simulink model "rolltesting"  (R2019a)
settings: Solver=VariableStepAuto  StartTime=0.0  StopTime=3  RelTol=1e-3
values from neighbouring files (symbols this model uses):
  D = zeros(size(B))    [RocketOutputFunction.m]    (also in StateSpaceController.m = zeros(13, 3); TimeDelayCompensationElevator.m = [0; 0])
  F = eye(6)    [MEKFAttitudeOnly.m]
  Ki2 = lqr(Ai2, Bi2, Q, R)    [StateSpaceController.m]
  q = x(13:16)    [AdaptiveLQR.m]    (also in MEKF.m = nominal_state(4:7); MEKFAttitudeOnly.m = [1 0 0 0]; MEKF_old.m = nominal_state(4:7); NonlinearStateEstimationForActuatorDelay.m = x(4:7))
  r = sym('r', [3 1])    [StateSpaceController.m]    (also in TimeDelayCompensationElevator.m = [0;0]; Tracker.m = [0; 0; -(rocket_length - Average_cg)])
  s = linspace(0, 100, nums)    [ImpactVelocityFunction.m]    (also in ImpactVelocityNotParallelMatlab.m = 1:5:500; ParallelImpactVelocity.m = .1:.01:500; ParralelRun.m = linspace(5,7, nums); RunImpactVelocityParforCompiled.m = 1:0.1:500)
undefined symbols (not defined in the file or in its folder): deg, e0_0, e1_0, e2_0, e3_0, Earth, Light, magnitude, MIL, rad, WGS84
libraries: aerolibutil x9, aerolibconvert2 x4, simulink x3, sharedtransform x3, aerolibwind2 x3, aerolibfltsims x2, aerolibasang x2, aerolibatmos2 x1, aerolibbdyn x1, aerolibtransform2 x1
settings Model: Creator=rag  LastModifiedBy=rag

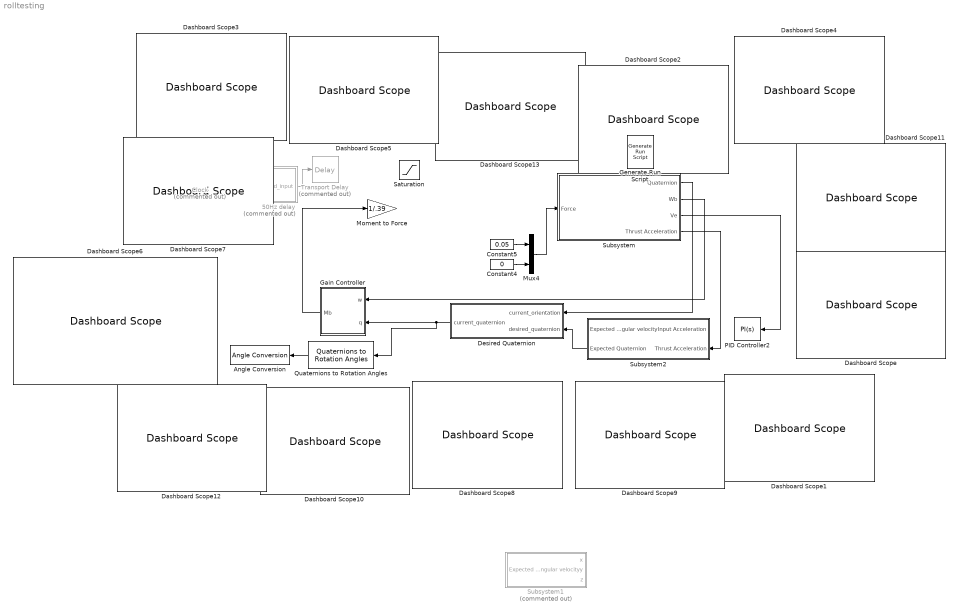
== system rolltesting ==
  50Hz delay : MATLAB Function  Commented=on  TreatAsAtomicUnit=on
  Angle Conversion : aerolibconvert2/Angle Conversion  IU=rad  OU=deg
  Clock : Clock  Commented=on
      settings: Decimation=100
  Constant4 : Constant  Value=0
  Constant5 : Constant  Value=0.05
  Dashboard Scope{,1..13} (14 alike) : DashboardScope
  Desired Quaternion : MATLAB Function  TreatAsAtomicUnit=on
  Gain Controller : Subsystem
  Generate Run Script : aerolibfltsims/Generate Run Script  Architecture=Win64  dataFlow=Send  GeometryModelName=Rocket  AirportId=PHNL  RunwayId=04L  InitialAltitude=13  InitialHeading=0  OffsetDistance=0  OffsetAzimuth=0  InstallScenery=off  DisableShaders=off  OriginAddress=127.0.0.1  DestinationPort=5502  OriginPort=5505  LocalAddress=127.0.0.1  OutputFileName=runfg.bat  FlightGearBaseDirectory=C:\Program Files\FlightGear 2018.2.2
  Moment to Force : Gain  Gain=1/.39
  Mux4 : Mux  Inputs=2
  PID Controller2 : simulink/Continuous/PID Controller  Controller=PI  Form=Parallel  TimeDomain=Continuous-time  SampleTime=-1  IntegratorMethod=Forward Euler  FilterMethod=Forward Euler  ControllerParametersSource=internal  P=-0.4  I=-0.3  D=0  UseFilter=on  N=100  TunerSelectOption=Transfer Function Based (PID Tuner App)  InitialConditionSource=internal  InitialConditionForIntegrator=0  InitialConditionForFilter=0  DifferentiatorICPrevScaledInput=0  ExternalReset=none  TrackingMode=off  Kt=1  LimitOutput=off  UpperSaturationLimit=inf  LowerSaturationLimit=-inf  LinearizeAsGain=on  AntiWindupMode=none  Kb=1  POutMin=[]  POutMax=[]  IOutMin=[]  IOutMax=[]  DOutMin=[]  DOutMax=[]  NOutMin=[]  NOutMax=[]  SumOutMin=[]  SumOutMax=[]  SaturationOutMin=[]  SaturationOutMax=[]  PParamMin=[]  PParamMax=[]  IParamMin=[]  IParamMax=[]  DParamMin=[]  DParamMax=[]  NParamMin=[]  NParamMax=[]  KbParamMin=[]  KbParamMax=[]  KtParamMin=[]  KtParamMax=[]  KbOutMin=[]  KbOutMax=[]  KtOutMin=[]  KtOutMax=[]  IntegratorOutMin=[]  IntegratorOutMax=[]  FilterOutMin=[]  FilterOutMax=[]  SumI1OutMin=[]  SumI1OutMax=[]  SumI2OutMin=[]  SumI2OutMax=[]  SumI3OutMin=[]  SumI3OutMax=[]  SumI4OutMin=[]  SumI4OutMax=[]  SumDOutMin=[]  SumDOutMax=[]  DifferentiatorOutMin=[]  DifferentiatorOutMax=[]  FilterDiffOutCoefMin=[]  FilterDiffOutCoefMax=[]  ReciprocalOutMin=[]  ReciprocalOutMax=[]  SumDenOutMin=[]  SumDenOutMax=[]  SumNumOutMin=[]  SumNumOutMax=[]  DivideOutMin=[]  DivideOutMax=[]  IntegratorContinuousStateAttributes=''  IntegratorStateMustResolveToSignalObject=off  IntegratorRTWStateStorageClass=Auto  FilterContinuousStateAttributes=''  FilterStateMustResolveToSignalObject=off  FilterRTWStateStorageClass=Auto  ParallelPVariant=InternalParameters  IdealPVariant=Disabled  IVariant=InternalParameters  DVariant=Disabled  IntegratorVariant=Continuous  SatVariant=Disabled  AWVariant=Passthrough  PCopyVariant=Disabled  TRVariant=Disabled  FdbkBlocksVariant=Forward  IdealPFdbkVariant=Disabled  SatFdbkVariant=Disabled  DerivativeFilterVariant=Disabled  NVariant=Disabled  NCopyVariant=Disabled_SignalSpec  FilterICVariant=Disabled  IntegratorICVariant=InternalICs  ExternalResetVariant=Disabled  TRSumVariant=Passthrough  SumFdbkVariant=Disabled  SumVariant=Sum_PI
  Quaternions to Rotation Angles : sharedtransform/Quaternions to Rotation Angles  rotationOrder=XYZ  aMode=aMode
      settings: SourceProductBaseCode=AE
  Saturation : Saturate  UpperLimit=1.5  LowerLimit=-1.5
  Subsystem : Subsystem
  Subsystem1 : Subsystem  Commented=on
  Subsystem2 : Subsystem
  Transport Delay : TransportDelay  Commented=on  DelayTime=0.015  TransDelayFeedthrough=on
  wires:
  Quaternions to Rotation Angles/1 -> Angle Conversion/1
  Desired Quaternion/1(current_quaternion) -> Quaternions to Rotation Angles/1, Gain Controller/2(q)
  Gain Controller/1(Mb) -> Moment to Force/1
  Subsystem/4(Thrust Acceleration) -> Subsystem2/2(Thrust Acceleration)
  50Hz delay/1(delayed_input) -> Transport Delay/1
  Subsystem/3(Ve) -> PID Controller2/1
  Subsystem/2(Wb) -> Gain Controller/1(w)
  Subsystem2/2(Expected Quaternion) -> Desired Quaternion/2(desired_quaternion)
  Clock/1 -> 50Hz delay/1(time)
  Subsystem/1(Quaternion) -> Desired Quaternion/1(current_orientation)
  Mux4/1 -> Subsystem/1(Force)
  Constant5/1 -> Mux4/1
  Constant4/1 -> Mux4/2

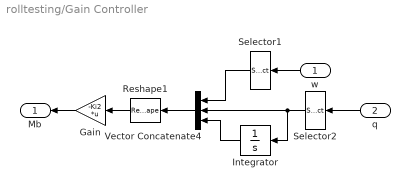
== system rolltesting/Gain Controller ==
  w : Inport
  q : Inport  Port=2
  Gain : Gain  Gain=-Ki2  Multiplication=Matrix(K*u)
  Integrator : Integrator
  Reshape1 : Reshape  OutputDimensionality=Column vector (2-D)
  Selector1 : Selector  InputPortWidth=3  IndexOptions=Index vector (dialog)  Indices=[2 1]  OutputSizes=1
  Selector2 : Selector  InputPortWidth=4  IndexOptions=Index vector (dialog)  Indices=[3 2]  OutputSizes=1
  Vector Concatenate4 : Concatenate  NumInputs=3
  Mb : Outport
  wires:
  Vector Concatenate4/1 -> Reshape1/1
  Reshape1/1 -> Gain/1
  Selector2/1 -> Integrator/1, Vector Concatenate4/2
  Integrator/1 -> Vector Concatenate4/3
  q/1 -> Selector2/1
  Gain/1 -> Mb/1
  Selector1/1 -> Vector Concatenate4/1
  w/1 -> Selector1/1

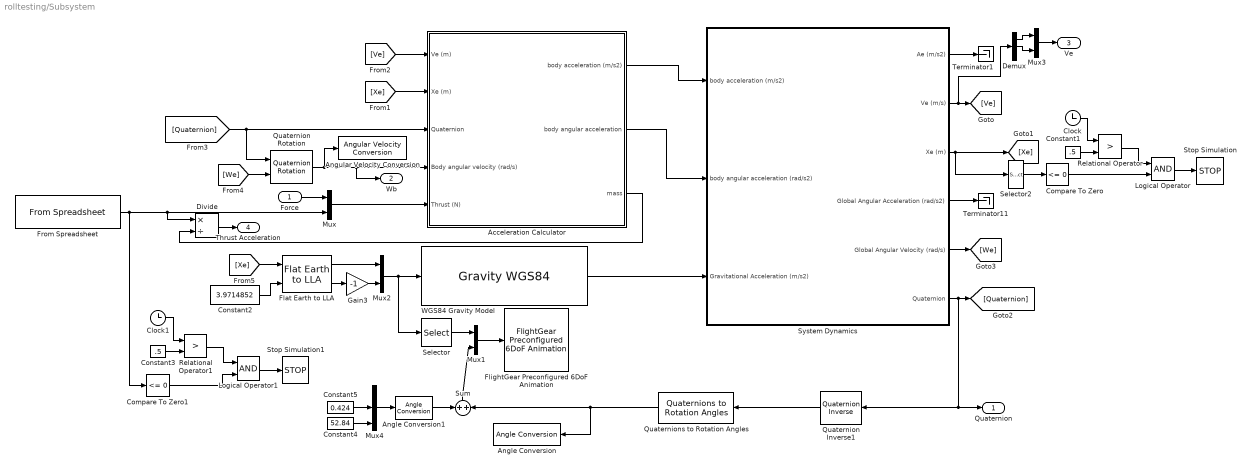
== system rolltesting/Subsystem ==
  Force : Inport  PortDimensions=2
  Acceleration Calculator : Subsystem
  Angle Conversion : aerolibconvert2/Angle Conversion  IU=rad  OU=deg
  Angle Conversion1 : aerolibconvert2/Angle Conversion  IU=deg  OU=rad
  Angular Velocity Conversion : aerolibconvert2/Angular Velocity Conversion  IU=rad/s  OU=deg/s
      settings: SourceProductName=Aerospace Blockset
  Clock : Clock
  Clock1 : Clock
  Compare To Zero : simulink/Logic and Bit Operations/Compare To Zero  relop=<=  OutDataTypeStr=boolean
  Compare To Zero1 : simulink/Logic and Bit Operations/Compare To Zero  relop=<=  OutDataTypeStr=boolean
  Constant1 : Constant  Value=.5
  Constant2 : Constant  Value=3.9714852
  Constant3 : Constant  Value=.5
  Constant4 : Constant  Value=52.84
  Constant5 : Constant  Value=0.424
  Demux : Demux  Outputs=3
  Divide : Product  Inputs=*/
  Flat Earth to LLA : aerolibtransform2/Flat Earth to LLA  units=Metric (MKS)  ptype=Earth (WGS84)  F=1/298.257223563  R=6378137  LL0=[21.318358277648 -157.9232805920725]  psi=052
  FlightGear Preconfigured 6DoF Animation : aerolibfltsims/FlightGear Preconfigured 6DoF Animation  xFlightGearVersion=v2018.2  DestinationIpAddress=127.0.0.1  DestinationPort=5502  SampleTime=1/100  packetVersion=24
      settings: SourceProductName=Aerospace Blockset
  From Spreadsheet : FromSpreadsheet  FileName=F10_Thrust.xls  Range=A1:B29  ExtrapolationBeforeFirstDataPoint=Hold first value  ExtrapolationAfterLastDataPoint=Hold last value
  Gain3 : Gain  Gain=-1
  Logical Operator : Logic  AllPortsSameDT=off  OutDataTypeStr=boolean
  Logical Operator1 : Logic  AllPortsSameDT=off  OutDataTypeStr=boolean
  Mux{,1..3} (4 alike) : Mux  Inputs=2
  Mux4 : Mux  Inputs=3
  Quaternion Inverse1 : aerolibutil/Quaternion Inverse
      settings: SourceProductName=Aerospace Blockset
  Quaternion Rotation : aerolibutil/Quaternion Rotation
  Quaternions to Rotation Angles : sharedtransform/Quaternions to Rotation Angles  rotationOrder=XYZ  aMode=aMode
      settings: SourceProductBaseCode=AE
  Relational Operator : RelationalOperator  Operator=>  OutDataTypeStr=boolean  RndMeth=Simplest
  Relational Operator1 : RelationalOperator  Operator=>  OutDataTypeStr=boolean  RndMeth=Simplest
  Selector : Selector  InputPortWidth=3  IndexOptions=Index vector (dialog)  Indices=[2 1 3]  OutputSizes=1
  Selector2 : Selector  InputPortWidth=3  IndexOptions=Index vector (dialog)  Indices=[3]  OutputSizes=1
  Stop Simulation : Stop
  Stop Simulation1 : Stop
  Sum : Sum
  System Dynamics : Subsystem
  Terminator1 : Terminator
  Terminator11 : Terminator
  "WGS84 Gravity Model  " : GravityWGS84
  Quaternion : Outport
  Wb : Outport  Port=2
  Ve : Outport  Port=3
  Thrust Acceleration : Outport  Port=4
  wires:
  System Dynamics/5(Global Angular Velocity (rad/s)) -> [We]
  Selector/1 -> Mux1/1
  [Quaternion] -> Quaternion Rotation/1, Acceleration Calculator/3(Quaternion)
  Flat Earth to LLA/1 -> Mux2/1
  Flat Earth to LLA/2 -> Gain3/1
  Mux/1 -> Acceleration Calculator/5(Thrust (N))
  Gain3/1 -> Mux2/2
  Quaternions to Rotation Angles/1 -> Sum/2, Angle Conversion/1
  Mux2/1 -> Selector/1, "WGS84 Gravity Model  "/1
  System Dynamics/2(Ve (m/s)) -> Demux/1, [Ve]
  Constant2/1 -> Flat Earth to LLA/2
  Acceleration Calculator/1(body acceleration (m/s2)) -> System Dynamics/1(body acceleration (m/s2))
  System Dynamics/6(Quaternion) -> Quaternion Inverse1/1, Quaternion/1, [Quaternion]
  From Spreadsheet/1 -> Compare To Zero1/1, Divide/1, Mux/2
  Quaternion Rotation/1 -> Angular Velocity Conversion/1, Wb/1, Acceleration Calculator/4(Body angular velocity (rad/s))
  [We] -> Quaternion Rotation/2
  [Ve] -> Acceleration Calculator/1(Ve (m))
  Mux1/1 -> FlightGear Preconfigured 6DoF Animation/1
  "WGS84 Gravity Model  "/1 -> System Dynamics/3(Gravitational Acceleration (m/s2))
  [Xe] -> Acceleration Calculator/2(Xe (m))
  Force/1 -> Mux/1
  System Dynamics/1(Ae (m/s2)) -> Terminator1/1
  System Dynamics/4(Global Angular Acceleration (rad/s2)) -> Terminator11/1
  Clock/1 -> Relational Operator/1
  Compare To Zero/1 -> Logical Operator/2
  Logical Operator/1 -> Stop Simulation/1
  Relational Operator/1 -> Logical Operator/1
  Constant1/1 -> Relational Operator/2
  Selector2/1 -> Compare To Zero/1
  Relational Operator1/1 -> Logical Operator1/1
  Logical Operator1/1 -> Stop Simulation1/1
  Constant3/1 -> Relational Operator1/2
  Clock1/1 -> Relational Operator1/1
  Compare To Zero1/1 -> Logical Operator1/2
  Demux/1 -> Mux3/1
  Demux/2 -> Mux3/2
  Mux3/1 -> Ve/1
  Constant4/1 -> Mux4/3
  Mux4/1 -> Angle Conversion1/1
  Constant5/1 -> Mux4/2
  Angle Conversion1/1 -> Sum/1
  [Xe] -> Flat Earth to LLA/1
  Sum/1 -> Mux1/2
  System Dynamics/3(Xe (m)) -> [Xe], Selector2/1
  Quaternion Inverse1/1 -> Quaternions to Rotation Angles/1
  Acceleration Calculator/3(mass) -> Divide/2
  Divide/1 -> Thrust Acceleration/1
  Acceleration Calculator/2(body angular acceleration) -> System Dynamics/2(body angular acceleration (rad/s2))

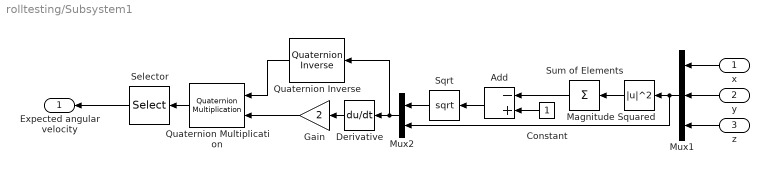
== system rolltesting/Subsystem1 ==
  x : Inport
  y : Inport  Port=2
  z : Inport  Port=3
  Add : Sum  Inputs=-+
  Constant : Constant
  Derivative : Derivative
  Gain : Gain  Gain=2
  Magnitude Squared : Math  Operator=magnitude^2  SaturateOnIntegerOverflow=on
  Mux1 : Mux  Inputs=3
  Mux2 : Mux  Inputs=2
  Quaternion Inverse : aerolibutil/Quaternion Inverse
      settings: SourceProductName=Aerospace Blockset
  Quaternion Multiplication : aerolibutil/Quaternion Multiplication
  Selector : Selector  InputPortWidth=4  IndexOptions=Index vector (dialog)  Indices=[2 3 4]  OutputSizes=1
  Sqrt : Sqrt  SaturateOnIntegerOverflow=on
  Sum of Elements : Sum  Inputs=+
  Expected angular velocity : Outport
  wires:
  Quaternion Inverse/1 -> Quaternion Multiplication/1
  x/1 -> Mux1/1
  Gain/1 -> Quaternion Multiplication/2
  Magnitude Squared/1 -> Sum of Elements/1
  Add/1 -> Sqrt/1
  Mux1/1 -> Mux2/2, Magnitude Squared/1
  Quaternion Multiplication/1 -> Selector/1
  Mux2/1 -> Quaternion Inverse/1, Derivative/1
  Constant/1 -> Add/2
  Derivative/1 -> Gain/1
  Sqrt/1 -> Mux2/1
  z/1 -> Mux1/3
  y/1 -> Mux1/2
  Sum of Elements/1 -> Add/1
  Selector/1 -> Expected angular velocity/1

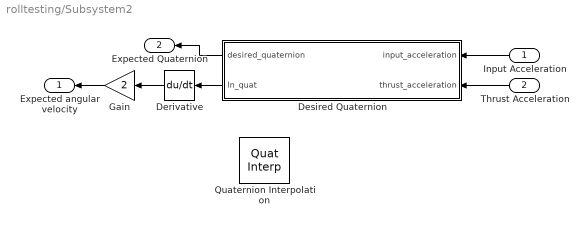
== system rolltesting/Subsystem2 ==
  Input Acceleration : Inport  PortDimensions=[2]
  Thrust Acceleration : Inport  Port=2
  Derivative : Derivative
  Desired Quaternion : MATLAB Function  TreatAsAtomicUnit=on
  Gain : Gain  Gain=2
  Quaternion Interpolation : QuatInterp
  Expected angular velocity : Outport
  Expected Quaternion : Outport  Port=2
  wires:
  Thrust Acceleration/1 -> Desired Quaternion/2(thrust_acceleration)
  Gain/1 -> Expected angular velocity/1
  Desired Quaternion/1(desired_quaternion) -> Expected Quaternion/1
  Input Acceleration/1 -> Desired Quaternion/1(input_acceleration)
  Derivative/1 -> Gain/1
  Desired Quaternion/2(ln_quat) -> Derivative/1

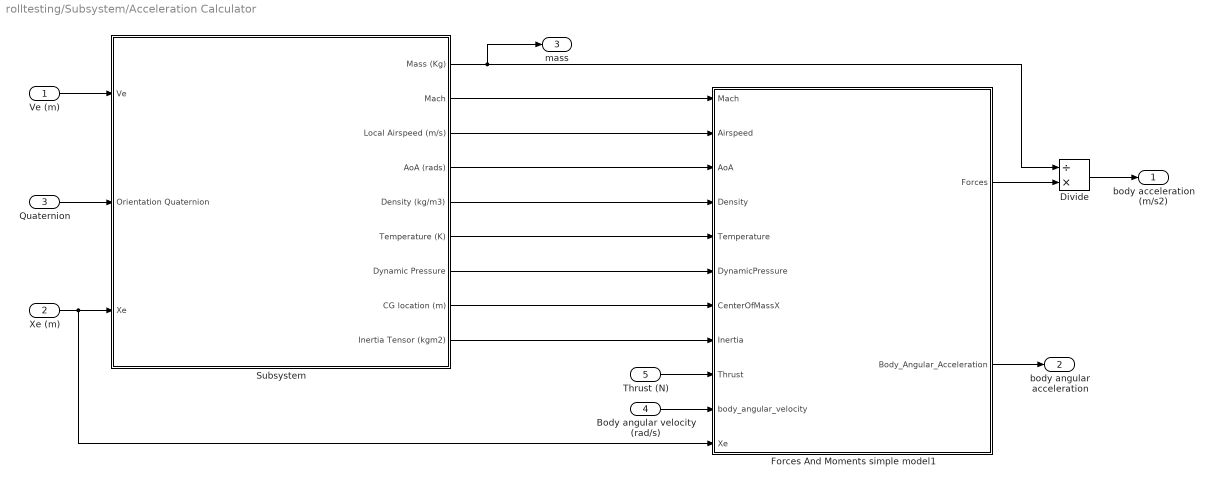
== system rolltesting/Subsystem/Acceleration Calculator ==
  Ve (m) : Inport
  Xe (m) : Inport  Port=2
  Quaternion : Inport  Port=3
  Body angular velocity (rad/s) : Inport  Port=4
  Thrust (N) : Inport  Port=5
  Divide : Product  Inputs=/*
  Forces And Moments simple model1 : MATLAB Function  TreatAsAtomicUnit=on
  Subsystem : Subsystem
  body acceleration (m/s2) : Outport
  body angular acceleration : Outport  Port=2
  mass : Outport  Port=3
  wires:
  Subsystem/4(AoA (rads)) -> Forces And Moments simple model1/3(AoA)
  Xe (m)/1 -> Forces And Moments simple model1/11(Xe), Subsystem/3(Xe)
  Subsystem/6(Temperature (K)) -> Forces And Moments simple model1/5(Temperature)
  Subsystem/8(CG location (m)) -> Forces And Moments simple model1/7(CenterOfMassX)
  Subsystem/3(Local Airspeed (m/s)) -> Forces And Moments simple model1/2(Airspeed)
  Subsystem/7(Dynamic Pressure) -> Forces And Moments simple model1/6(DynamicPressure)
  Subsystem/2(Mach) -> Forces And Moments simple model1/1(Mach)
  Subsystem/5(Density (kg/m3)) -> Forces And Moments simple model1/4(Density)
  Thrust (N)/1 -> Forces And Moments simple model1/9(Thrust)
  Forces And Moments simple model1/1(Forces) -> Divide/2
  Body angular velocity (rad/s)/1 -> Forces And Moments simple model1/10(body_angular_velocity)
  Ve (m)/1 -> Subsystem/1(Ve)
  Quaternion/1 -> Subsystem/2(Orientation Quaternion)
  Subsystem/9(Inertia Tensor (kgm2)) -> Forces And Moments simple model1/8(Inertia)
  Forces And Moments simple model1/2(Body_Angular_Acceleration) -> body angular acceleration/1
  Divide/1 -> body acceleration (m/s2)/1
  Subsystem/1(Mass (Kg)) -> mass/1, Divide/1

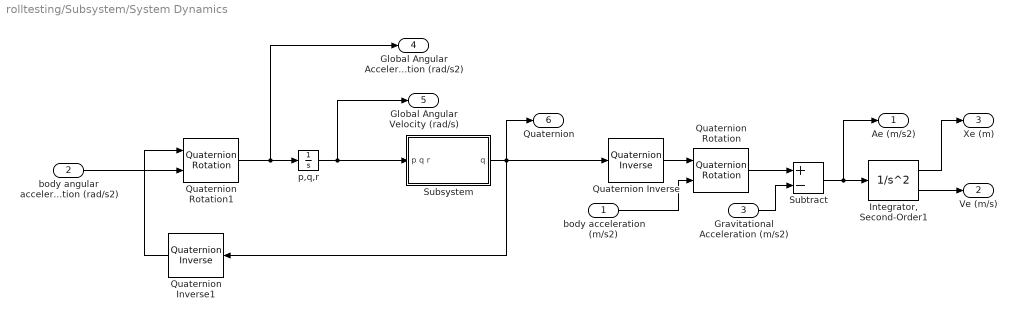
== system rolltesting/Subsystem/System Dynamics ==
  body acceleration (m/s2) : Inport  Unit=N*m  PortDimensions=3
  body angular acceleration (rad/s2) : Inport  Port=2  PortDimensions=3
  Gravitational Acceleration (m/s2) : Inport  Port=3
  "Integrator, Second-Order1" : SecondOrderIntegrator  LimitX=on  LowerLimitX=[-inf; -inf; 0]
  Quaternion Inverse : aerolibutil/Quaternion Inverse
      settings: SourceProductName=Aerospace Blockset
  Quaternion Inverse1 : aerolibutil/Quaternion Inverse
      settings: SourceProductName=Aerospace Blockset
  Quaternion Rotation : aerolibutil/Quaternion Rotation
  Quaternion Rotation1 : aerolibutil/Quaternion Rotation
  Subsystem : Subsystem
  Subtract : Sum  Inputs=+-
  "p,q,r " : Integrator
  Ae (m/s2) : Outport  Unit=m/s^2
  Ve (m/s) : Outport  Port=2  Unit=m/s
  Xe (m) : Outport  Port=3  Unit=m
  Global Angular Acceleration (rad/s2) : Outport  Port=4  Unit=rad/s
  Global Angular Velocity (rad/s) : Outport  Port=5  Unit=rad/s
  Quaternion : Outport  Port=6  Unit=1
  wires:
  "p,q,r "/1 -> Subsystem/1(p q r), Global Angular Velocity (rad/s)/1
  body acceleration (m/s2)/1 -> Quaternion Rotation/2
  Subsystem/1(q) -> Quaternion/1, Quaternion Inverse/1, Quaternion Inverse1/1
  Quaternion Inverse/1 -> Quaternion Rotation/1
  "Integrator, Second-Order1"/1 -> Xe (m)/1
  Gravitational Acceleration (m/s2)/1 -> Subtract/2
  Quaternion Rotation/1 -> Subtract/1
  "Integrator, Second-Order1"/2 -> Ve (m/s)/1
  Subtract/1 -> "Integrator, Second-Order1"/1, Ae (m/s2)/1
  Quaternion Inverse1/1 -> Quaternion Rotation1/1
  body angular acceleration (rad/s2)/1 -> Quaternion Rotation1/2
  Quaternion Rotation1/1 -> Global Angular Acceleration (rad/s2)/1, "p,q,r "/1

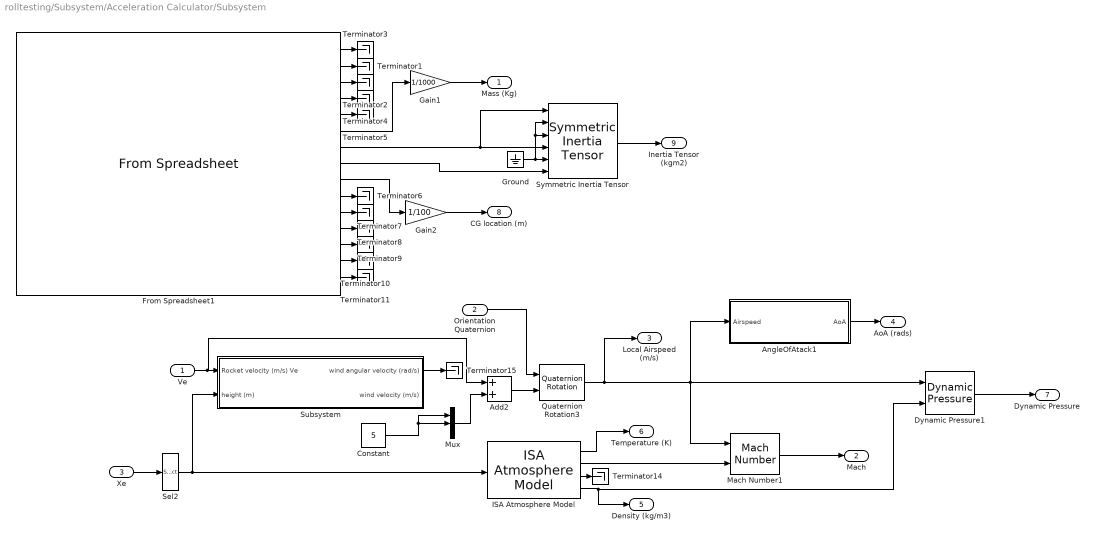
== system rolltesting/Subsystem/Acceleration Calculator/Subsystem ==
  Ve : Inport
  Orientation Quaternion : Inport  Port=2
  Xe : Inport  Port=3
  Add2 : Sum
  AngleOfAtack1 : MATLAB Function  TreatAsAtomicUnit=on
  Constant : Constant  Value=5
  Dynamic Pressure1 : aerolibasang/Dynamic Pressure
  From Spreadsheet1 : FromSpreadsheet  FileName=C:\Users\rag\Documents\GitHub\EPQ\OpenRocket\bodyacceleraiton.xlsx  SheetName=bodyacceleraiton  Range=A1:P4395  ExtrapolationBeforeFirstDataPoint=Hold first value  ExtrapolationAfterLastDataPoint=Hold last value
  Gain1 : Gain  Gain=1/1000
  Gain2 : Gain  Gain=1/100
  Ground : Ground
  ISA Atmosphere Model : aerolibatmos2/ISA Atmosphere Model  custom=on  g=9.80665  gamma=1.4  R=287.0531  L=0.0065  h_trop=11000  h_strat=20000  rho0=1.225  P0=Pressure  T0=Temperature  h0=0
      settings: SourceProductName=Aerospace Blockset
  Mach Number1 : aerolibasang/Mach Number
      settings: SourceProductName=Aerospace Blockset  SourceProductBaseCode=AE
  Mux : Mux  Inputs=3
  Quaternion Rotation3 : aerolibutil/Quaternion Rotation
  Sel2 : Selector  InputPortWidth=3  IndexOptions=Index vector (dialog)  Indices=3  OutputSizes=1
  Subsystem : Subsystem
  Symmetric Inertia Tensor : aerolibbdyn/Symmetric Inertia Tensor
      settings: SourceProductName=Aerospace Blockset  SourceProductBaseCode=AE
  Terminator{1..11,14..15} (13 alike) : Terminator
  Mass (Kg) : Outport
  Mach : Outport  Port=2
  Local Airspeed (m/s) : Outport  Port=3
  AoA (rads) : Outport  Port=4
  Density (kg/m3) : Outport  Port=5
  Temperature (K) : Outport  Port=6
  Dynamic Pressure : Outport  Port=7
  CG location (m) : Outport  Port=8
  Inertia Tensor (kgm2) : Outport  Port=9
  wires:
  From Spreadsheet1/8 -> Symmetric Inertia Tensor/6
  From Spreadsheet1/4 -> Terminator4/1
  Quaternion Rotation3/1 -> Local Airspeed (m/s)/1, AngleOfAtack1/1(Airspeed), Dynamic Pressure1/1, Mach Number1/1
  ISA Atmosphere Model/4 -> Density (kg/m3)/1, Dynamic Pressure1/2
  Add2/1 -> Quaternion Rotation3/2
  From Spreadsheet1/5 -> Terminator5/1
  From Spreadsheet1/9 -> Gain2/1
  From Spreadsheet1/6 -> Gain1/1
  ISA Atmosphere Model/2 -> Mach Number1/2
  ISA Atmosphere Model/1 -> Temperature (K)/1
  Dynamic Pressure1/1 -> Dynamic Pressure/1
  Orientation Quaternion/1 -> Quaternion Rotation3/1
  Mach Number1/1 -> Mach/1
  From Spreadsheet1/12 -> Terminator8/1
  AngleOfAtack1/1(AoA) -> AoA (rads)/1
  ISA Atmosphere Model/3 -> Terminator14/1
  Gain2/1 -> CG location (m)/1
  From Spreadsheet1/7 -> Symmetric Inertia Tensor/1, Symmetric Inertia Tensor/4
  From Spreadsheet1/11 -> Terminator7/1
  Xe/1 -> Sel2/1
  From Spreadsheet1/3 -> Terminator2/1
  From Spreadsheet1/14 -> Terminator10/1
  From Spreadsheet1/2 -> Terminator1/1
  From Spreadsheet1/1 -> Terminator3/1
  From Spreadsheet1/13 -> Terminator9/1
  From Spreadsheet1/15 -> Terminator11/1
  Gain1/1 -> Mass (Kg)/1
  Ground/1 -> Symmetric Inertia Tensor/2, Symmetric Inertia Tensor/3, Symmetric Inertia Tensor/5
  Symmetric Inertia Tensor/1 -> Inertia Tensor (kgm2)/1
  From Spreadsheet1/10 -> Terminator6/1
  Subsystem/1(wind angular velocity (rad/s)) -> Terminator15/1
  Ve/1 -> Add2/1, Subsystem/1(Rocket velocity (m/s) Ve)
  Sel2/1 -> Subsystem/2(height (m)), ISA Atmosphere Model/1
  Mux/1 -> Add2/2
  Constant/1 -> Mux/2, Mux/1

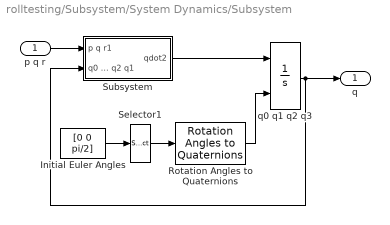
== system rolltesting/Subsystem/System Dynamics/Subsystem ==
  p q r : Inport
  Initial Euler Angles : Constant  Value=[0 0 pi/2]
  Rotation Angles to Quaternions : sharedtransform/Rotation Angles to Quaternions  rotationOrder=ZYX  aMode=aMode
      settings: SourceProductName=Aerospace Blockset  SourceProductBaseCode=AE
  Selector1 : Selector  InputPortWidth=3  IndexOptions=Index vector (dialog)  Indices=[3 2 1]  OutputSizes=1
  Subsystem : Subsystem
  q0 q1 q2 q3 : Integrator  InitialConditionSource=external  InitialCondition=[e0_0 e1_0 e2_0 e3_0]
  q : Outport
  wires:
  Rotation Angles to Quaternions/1 -> q0 q1 q2 q3/2
  Initial Euler Angles/1 -> Selector1/1
  Subsystem/1(qdot2) -> q0 q1 q2 q3/1
  Selector1/1 -> Rotation Angles to Quaternions/1
  p q r/1 -> Subsystem/1(p q r1)
  q0 q1 q2 q3/1 -> q/1, Subsystem/2(q0 q1 q2 q1)

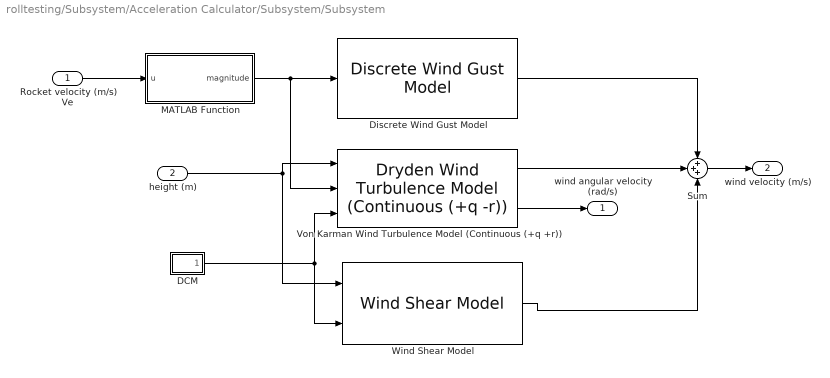
== system rolltesting/Subsystem/Acceleration Calculator/Subsystem/Subsystem ==
  Rocket velocity (m/s) Ve : Inport
  height (m) : Inport  Port=2
  DCM : MATLAB Function  TreatAsAtomicUnit=on
  Discrete Wind Gust Model : aerolibwind2/Discrete Wind Gust Model  units=Metric (MKS)  Gx=on  Gy=on  Gz=on  t_0=GustStart  d_m=GustLength  v_m=GuestAmplitude
      settings: SourceProductName=Aerospace Blockset
  MATLAB Function : MATLAB Function  TreatAsAtomicUnit=on
  Sum : Sum  Inputs=3
  Von Karman Wind Turbulence Model (Continuous (+q +r)) : aerolibwind2/Dryden Wind Turbulence Model  (Continuous (+q -r))  units=Metric (MKS)  spec=MIL-F-8785C  model=Discrete Dryden (+q -r)  W20=ShearSpeed  Wdeg=ShearDirection  TurbProb=10^-2 - Light  L_high=762  Wingspan=10  ts=0.1  Seed=[23341 23342 23343 23344]  T_on=on
      settings: SourceProductName=Aerospace Blockset
  Wind Shear Model : aerolibwind2/Wind Shear Model  units=Metric (MKS)  phase=Category C - Terminal Flight Phase  W_20=ShearSpeed  Wdeg=ShearDirection
      settings: SourceProductName=Aerospace Blockset
  wind angular velocity (rad/s) : Outport
  wind velocity (m/s) : Outport  Port=2
  wires:
  height (m)/1 -> Wind Shear Model/1, Von Karman Wind Turbulence Model (Continuous (+q +r))/1
  Discrete Wind Gust Model/1 -> Sum/1
  DCM/1(DCM) -> Von Karman Wind Turbulence Model (Continuous (+q +r))/3, Wind Shear Model/2
  MATLAB Function/1(magnitude) -> Von Karman Wind Turbulence Model (Continuous (+q +r))/2, Discrete Wind Gust Model/1
  Sum/1 -> wind velocity (m/s)/1
  Wind Shear Model/1 -> Sum/3
  Von Karman Wind Turbulence Model (Continuous (+q +r))/1 -> Sum/2
  Von Karman Wind Turbulence Model (Continuous (+q +r))/2 -> wind angular velocity (rad/s)/1
  Rocket velocity (m/s) Ve/1 -> MATLAB Function/1(u)

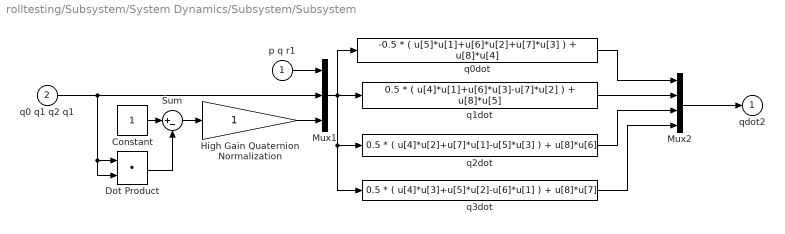
== system rolltesting/Subsystem/System Dynamics/Subsystem/Subsystem ==
  p q r1 : Inport
  q0 q1 q2 q1 : Inport  Port=2
  Constant : Constant
  Dot Product : DotProduct  OutDataTypeStr=Inherit: Inherit via internal rule
  High Gain Quaternion Normalization : Gain  SaturateOnIntegerOverflow=on  OutDataTypeStr=Inherit: Same as input  ParamDataTypeStr=Inherit: Same as input
  Mux1 : Mux  Inputs=[3 4 1]
  Mux2 : Mux
  Sum : Sum  Inputs=|+-  SaturateOnIntegerOverflow=on  InputSameDT=on  OutDataTypeStr=Inherit: Same as first input
  q0dot : Fcn  Expr=-0.5 * ( u[5]*u[1]+u[6]*u[2]+u[7]*u[3] ) + u[8]*u[4]
  q1dot : Fcn  Expr=0.5 * ( u[4]*u[1]+u[6]*u[3]-u[7]*u[2] ) + u[8]*u[5]
  q2dot : Fcn  Expr=0.5 * ( u[4]*u[2]+u[7]*u[1]-u[5]*u[3] ) + u[8]*u[6]
  q3dot : Fcn  Expr=0.5 * ( u[4]*u[3]+u[5]*u[2]-u[6]*u[1] ) + u[8]*u[7]
  qdot2 : Outport  InitialOutput=0
  wires:
  q0 q1 q2 q1/1 -> Dot Product/1, Dot Product/2, Mux1/2
  Mux1/1 -> q2dot/1, q3dot/1, q0dot/1, q1dot/1
  Constant/1 -> Sum/1
  High Gain Quaternion Normalization/1 -> Mux1/3
  q1dot/1 -> Mux2/2
  q0dot/1 -> Mux2/1
  Sum/1 -> High Gain Quaternion Normalization/1
  Dot Product/1 -> Sum/2
  q3dot/1 -> Mux2/4
  Mux2/1 -> qdot2/1
  q2dot/1 -> Mux2/3
  p q r1/1 -> Mux1/1

== matlab function rolltesting/50Hz delay ==
  settings: updateMethod=DISCRETE
  data: time input; input input; delayed_input output
function delayed_input = Servo(time, input)
    persistent lastupdate
    if isempty(lastupdate)
        lastupdate = [0;0];
    end
    
    servo_frequency = 50; %Hz
    if mod(time, 1/servo_frequency) == 0
        lastupdate = input;
    end    
        
    delayed_input = lastupdate;
end

== matlab function rolltesting/Subsystem/Acceleration Calculator/Subsystem/AngleOfAtack1 ==
  settings: updateMethod=DISCRETE
  data: Airspeed input; AoA output
function AoA = AngleOfAttack(Airspeed)
    AoA = acos(Airspeed(3) / norm(Airspeed));
        
    if norm(Airspeed) <= .01
        AoA = 0;
    end
end

== matlab function rolltesting/Subsystem/Acceleration Calculator/Forces And Moments simple model1 ==
  settings: updateMethod=DISCRETE
  data: Mach input; Airspeed input size=[3 1]; AoA input; Density input; Temperature input; DynamicPressure input; CenterOfMassX input; Inertia input; Thrust input; Forces output; body_angular_velocity input; Xe input; Body_Angular_Acceleration output
function [Forces, Body_Angular_Acceleration]  = forces(Mach, Airspeed, AoA, Density, Temperature, DynamicPressure, CenterOfMassX, Inertia, Thrust, body_angular_velocity, Xe)
    persistent ThetaRotation
    if isempty(ThetaRotation)
         ThetaRotation = eye(3);
    end
    
    %% Rocket Shape Constants
    Reference_Diameter = 7.62e-2;
    Reference_Radius = Reference_Diameter / 2;
    Reference_Area = Reference_Radius^2 * pi;
    
    NoseCone_Length = 15e-2;
    BodyTube_Length = 80e-2; 
    NoseCone_WetArea = pi * Reference_Radius * NoseCone_Length;          % pi*r*l 
    BodyTube_WetArea = pi * Reference_Radius * 2 * BodyTube_Length;      % pi*d*l
    NoseCone_PlanformArea = Reference_Diameter * NoseCone_Length / 2;
    BodyTube_PlanformArea = Reference_Diameter * BodyTube_Length;
    
    SurfaceRoughness = 20e-6;
    
    sinphi = Reference_Radius / hypot(Reference_Radius, NoseCone_Length);
    BodyTube_CP = 0.55;
    NoseCone_CP = 0.1;
    PitchCenterX = 0;
   
    
    COT_to_COM = .95 - CenterOfMassX; %get actual value and change over time as solid motor burns
    
    %% General Constants
    K = 1.1;
   
    %% Coefficients
    angularrate_local = ThetaRotation \ body_angular_velocity;
    [CN, Cpitch] = CalculatePitchAndNormalCDs(Mach, K, Reference_Diameter, AoA, Airspeed, angularrate_local(2), NoseCone_Length, BodyTube_Length, Reference_Area, CenterOfMassX, PitchCenterX, NoseCone_PlanformArea, BodyTube_PlanformArea, NoseCone_CP, BodyTube_CP);

    Cbase = .12 + .13*Mach^2;
    CFrictionDrag = CalculateFrictionDrag(Temperature, Density, Reference_Radius, Reference_Area, SurfaceRoughness, NoseCone_Length, BodyTube_Length, Airspeed, Mach, NoseCone_WetArea, BodyTube_WetArea);
    Cpressure = PressureDragForce(sinphi);
    
    Cdrag = Cbase + CFrictionDrag + Cpressure;
    Caxial = AxialDragMul(AoA) * Cdrag;

    Cyaw = 0.0;
    Croll = 0 * (rand - 0.5);
    Cside = 0;
    
     %% Random Noise to pitch and yaw coefficients in the range of +- 5e-4
    Cpitch = Cpitch + .1 * (rand - 0.5);
    Cyaw = Cyaw + .1 * (rand - 0.5);
    Croll = Croll + .1 * (rand - 0.5);
    %% Forces and Moments
    lengtha = norm(Airspeed(1:2));  
    
    sina = Airspeed(2) / lengtha;
    cosa = Airspeed(1) / lengtha;

    ThetaRotation = [cosa, -sina, 0; sina, cosa, 0; 0, 0, 1];
    
    z = DynamicPressure * Reference_Area;
    Thrust_moment = COT_to_COM * [Thrust(2); Thrust(1); 0];

    Forces = ThetaRotation * (Thrust + z * -[CN; Cside; Caxial]);
    Moments = [0; 0; 0] + Thrust_moment;
    
    if Xe(3) <= 0
        Forces = [0;0;Forces(3)];
        Moments = [0; 0; 0];
    end
    
    Body_Angular_Acceleration = Inertia \ Moments;
end

== matlab function rolltesting/Subsystem2/Desired Quaternion ==
  settings: updateMethod=DISCRETE
  data: input_acceleration input; thrust_acceleration input; desired_quaternion output size=[1 4]; ln_quat output
function [desired_quaternion, ln_quat] = func(input_acceleration, thrust_acceleration)

    max_horizontal_acceleration = sin(pi/12) * thrust_acceleration;
    if norm(input_acceleration) > max_horizontal_acceleration
        input_acceleration = input_acceleration * max_horizontal_acceleration / norm(input_acceleration);
    end
    
    global_thrust = [input_acceleration.', (thrust_acceleration^2 - norm(input_acceleration)^2)^.5];
    
    if norm(global_thrust) == 0
        global_thrust = [0,0,1];
    end
    
    desired_quaternion = quatnormalize([ global_thrust(3) + norm(global_thrust), cross([0;0;1], global_thrust) ]);
    
    if norm(desired_quaternion(2:4)) == 0
        ln_quat = [0 0 0];
    else
        ln_quat = desired_quaternion(2:4)/norm(desired_quaternion(2:4)) * desired_quaternion(1);
    end

== matlab function rolltesting/Desired Quaternion ==
  settings: updateMethod=DISCRETE
  data: current_orientation input; desired_quaternion input; current_quaternion output size=[1 4]
function current_quaternion = func(current_orientation, desired_quaternion)
    current_quaternion = quatmultiply(desired_quaternion, quatinv(current_orientation.')); %rotate to identity quat then to desired orientation 
    
    theta = atan( current_quaternion(4) / current_quaternion(1) ); %half the roll angle
    roll = [cos(theta), 0, 0, sin(theta)]; %extract roll part of quaternion
    current_quaternion = quatmultiply(current_quaternion, quatinv(roll)); %remove roll component
    
    current_quaternion = quatinv( current_quaternion); % then take the inverse to pretend to be at inverse orientation, due to state space being designed like that

== matlab function rolltesting/Subsystem/Acceleration Calculator/Subsystem/Subsystem/DCM ==
  settings: updateMethod=DISCRETE
  data: DCM output
function DCM  = forces
    DCM = [1,0,0;0,1,0;0,0,1];

== matlab function rolltesting/Subsystem/Acceleration Calculator/Subsystem/Subsystem/MATLAB Function ==
  data: u input; magnitude output
function magnitude = VectorNorm(u)
    magnitude = norm(u);
